simulink model "SIM_continuousFermenter"  (R2023b)
settings: Solver=VariableStepAuto  StartTime=0.0  StopTime=500  RelTol=1e-3
values from neighbouring files (symbols this model uses):
  Ts = 0.5    [NMPC_conFer.m]
libraries: sharedTrackingLibrary x1, mpclib x1, simulink x1, SignalEditorBlockLib x1
settings Model: Creator=akeebismail  LastModifiedBy=akeebismail

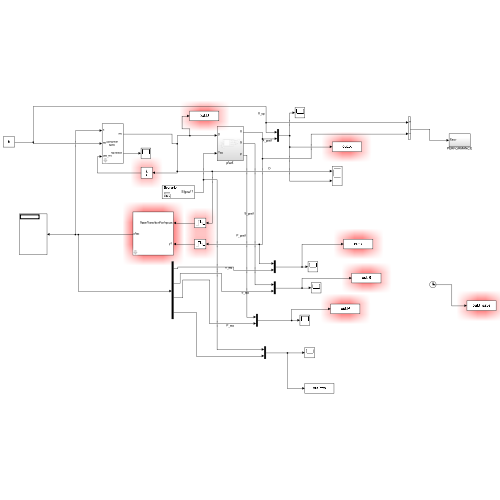
[thumbnail: Simulink's stored preview of the top-level diagram]
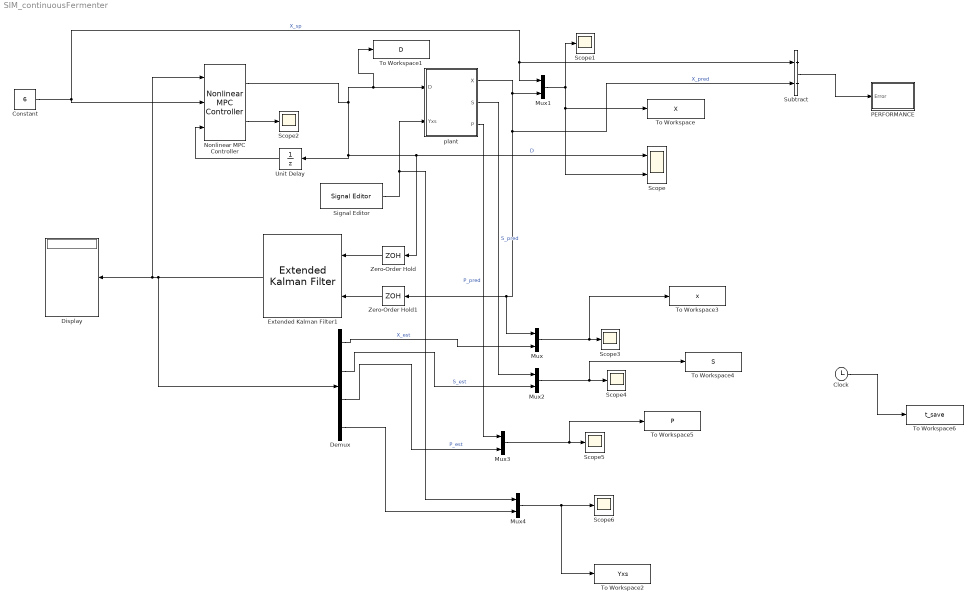
== system SIM_continuousFermenter ==
  Clock : Clock
  Constant : Constant  Value=6
  Demux : Demux
  Display : Display
  Extended Kalman Filter1 : sharedTrackingLibrary/Extended Kalman Filter  StateTransitionFcn=conFerStateFcnDT  HasStateTransitionJacobianFcn=off  HasAdditiveProcessNoise=Additive  ProcessNoise=[1e1;1e1;1e1;0.2]  HasTimeVaryingProcessNoise=off  HasStateTransitionFcnExtraArgument=1  InitialState=x0  InitialStateCovariance=[1;1;1;1]  MeasurementFcn1=conFerMeasFcn  HasMeasurementJacobianFcn1=off  HasMeasurementEnablePort1=off  HasAdditiveMeasurementNoise1=Additive  MeasurementNoise1=1e-3  HasTimeVaryingMeasurementNoise1=off  HasMeasurementFcnExtraArgument1=0  HasMeasurementWrapping1=off  MeasurementFcn2=myMeasurementFcn  HasMeasurementJacobianFcn2=off  HasMeasurementEnablePort2=off  HasAdditiveMeasurementNoise2=Additive  MeasurementNoise2=1  HasTimeVaryingMeasurementNoise2=off  HasMeasurementFcnExtraArgument2=0  HasMeasurementWrapping2=off  MeasurementFcn3=myMeasurementFcn  HasMeasurementJacobianFcn3=off  HasMeasurementEnablePort3=off  HasAdditiveMeasurementNoise3=Additive  MeasurementNoise3=1  HasTimeVaryingMeasurementNoise3=off  HasMeasurementFcnExtraArgument3=0  HasMeasurementWrapping3=off  MeasurementFcn4=myMeasurementFcn  HasMeasurementJacobianFcn4=off  HasMeasurementEnablePort4=off  HasAdditiveMeasurementNoise4=Additive  MeasurementNoise4=1  HasTimeVaryingMeasurementNoise4=off  HasMeasurementFcnExtraArgument4=0  HasMeasurementWrapping4=off  MeasurementFcn5=myMeasurementFcn  HasMeasurementJacobianFcn5=off  HasMeasurementEnablePort5=off  HasAdditiveMeasurementNoise5=Additive  MeasurementNoise5=1  HasTimeVaryingMeasurementNoise5=off  HasMeasurementFcnExtraArgument5=0  HasMeasurementWrapping5=off  EnableMultirate=off  StateTransitionFcnSampleTime=1  MeasurementFcn1SampleTime=1  MeasurementFcn2SampleTime=1  MeasurementFcn3SampleTime=1  MeasurementFcn4SampleTime=1  MeasurementFcn5SampleTime=1  UseCurrentEstimator=on  OutputStateCovariance=off  DataType=double  SampleTime=Ts  NumberOfMeasurements=1
  Mux{,1..4} (5 alike) : Mux  Inputs=2
  Nonlinear MPC Controller : mpclib/Nonlinear MPC Controller  nlmpcobj=nlobj  UseObjectTs=on  UseMEX=off  md_enabled=off  mvtarget_enabled=off  param_enabled=off  cost_enabled=off  mvseq_enabled=off  stateseq_enabled=off  ovseq_enabled=off  slack_enabled=off  status_enabled=on  ov_min=off  ov_max=off  mv_min=off  mv_max=off  mvrate_min=off  mvrate_max=off  state_min=off  state_max=off  ov_weight=off  mv_weight=off  mvrate_weight=off  ecr_weight=off  nlp_initialize=off
  PERFORMANCE : Subsystem
  Scope : Scope  NumInputPorts=2
  Scope{1..6} (6 alike) : Scope
  Signal Editor : SignalEditorBlockLib/Signal Editor  FileName=Yxs.mat  ActiveScenario=Scenario  ActiveSignal=Signal 1  IsBus=off  OutputBusObjectStr=Bus: BusObject  SampleTime=Ts  Interpolate=off  ZeroCross=off  OutputAfterFinalValue=Setting to zero  Unit=inherit  PreserveSignalName=on  ApplySigPropsToAllScenarios=on  ApplySigPropsToAllSignals=off
  Subtract : Sum  Inputs=+-
  To Workspace : ToWorkspace  VariableName=X  SaveFormat=Timeseries  SampleTime=Ts
  To Workspace1 : ToWorkspace  VariableName=D  SaveFormat=Timeseries  SampleTime=Ts
  To Workspace2 : ToWorkspace  VariableName=Yxs  SaveFormat=Timeseries  SampleTime=-1
  To Workspace3 : ToWorkspace  VariableName=x  SaveFormat=Timeseries  SampleTime=Ts
  To Workspace4 : ToWorkspace  VariableName=S  SaveFormat=Timeseries  SampleTime=Ts
  To Workspace5 : ToWorkspace  VariableName=P  SaveFormat=Timeseries  SampleTime=Ts
  To Workspace6 : ToWorkspace  VariableName=t_save  SaveFormat=Timeseries  SampleTime=Ts
  Unit Delay : UnitDelay  InitialCondition=0.202  SampleTime=Ts  HasFrameUpgradeWarning=on
  Zero-Order Hold : ZeroOrderHold  SampleTime=Ts
  Zero-Order Hold1 : ZeroOrderHold  SampleTime=Ts
  plant : Subsystem
  wires:
  Nonlinear MPC Controller/1 -> Zero-Order Hold/1, Scope/1, Unit Delay/1, To Workspace1/1, plant/1(D)  "D"
  Constant/1 -> Nonlinear MPC Controller/2, Subtract/1, Mux1/1  "X_sp"
  Nonlinear MPC Controller/2 -> Scope2/1
  plant/1(X) -> Subtract/2, Zero-Order Hold1/1, Mux/1, Mux1/2  "X_pred"
  Unit Delay/1 -> Nonlinear MPC Controller/3
  Mux1/1 -> Scope/2, To Workspace/1, Scope1/1
  Extended Kalman Filter1/1 -> Demux/1, Nonlinear MPC Controller/1, Display/1
  Zero-Order Hold/1 -> Extended Kalman Filter1/1
  Mux/1 -> To Workspace3/1, Scope3/1
  Demux/1 -> Mux/2  "X_est"
  Zero-Order Hold1/1 -> Extended Kalman Filter1/2
  Demux/3 -> Mux3/2  "P_est"
  Demux/2 -> Mux2/2  "S_est"
  plant/2(S) -> Mux2/1  "S_pred"
  plant/3(P) -> Mux3/1  "P_pred"
  Mux2/1 -> To Workspace4/1, Scope4/1
  Mux3/1 -> To Workspace5/1, Scope5/1
  Demux/4 -> Mux4/2
  Signal Editor/1 -> Mux4/1, plant/2(Yxs)
  Mux4/1 -> To Workspace2/1, Scope6/1
  Clock/1 -> To Workspace6/1
  Subtract/1 -> PERFORMANCE/1(Error)

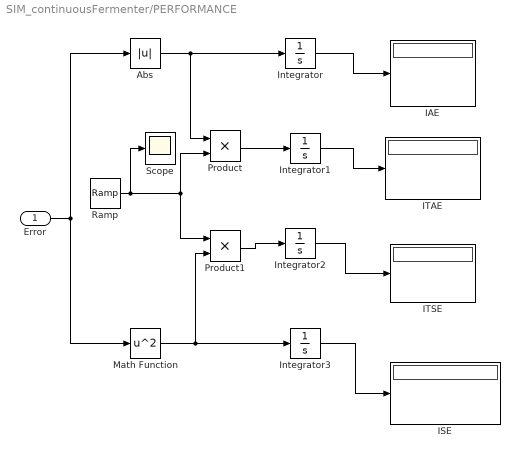
== system SIM_continuousFermenter/PERFORMANCE ==
  Error : Inport
  Abs : Abs  SaturateOnIntegerOverflow=off
  IAE : Display
  ISE : Display
  ITAE : Display
  ITSE : Display
  Integrator{,1..3} (4 alike) : Integrator
  Math Function : Math  Operator=square  SignedPower=on
  Product : Product  RndMeth=Zero
  Product1 : Product  RndMeth=Zero
  Ramp : simulink/Sources/Ramp  slope=1  start=0  InitialOutput=0
  Scope : Scope
  wires:
  Error/1 -> Math Function/1, Abs/1
  Abs/1 -> Integrator/1, Product/1
  Integrator/1 -> IAE/1
  Ramp/1 -> Product/2, Product1/1, Scope/1
  Math Function/1 -> Integrator3/1, Product1/2
  Product1/1 -> Integrator2/1
  Product/1 -> Integrator1/1
  Integrator3/1 -> ISE/1
  Integrator2/1 -> ITSE/1
  Integrator1/1 -> ITAE/1

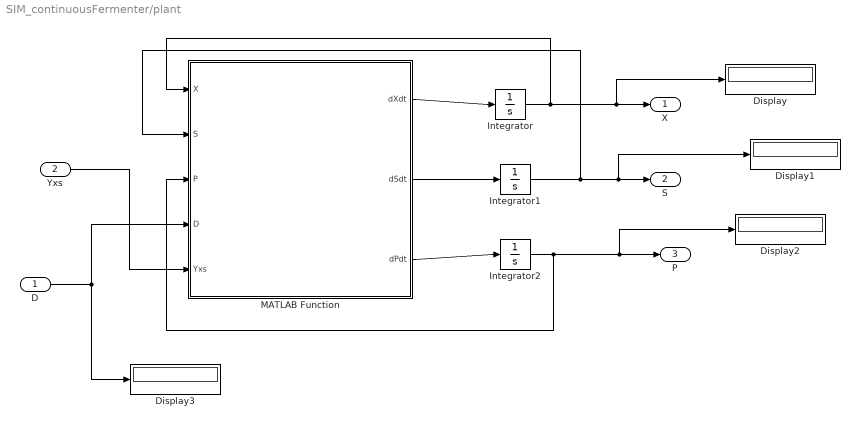
== system SIM_continuousFermenter/plant ==
  D : Inport
  Yxs : Inport  Port=2
  Display{,1..3} (4 alike) : Display
  Integrator : Integrator  InitialCondition=5
  Integrator1 : Integrator  InitialCondition=5
  Integrator2 : Integrator  InitialCondition=19.14
  MATLAB Function : MATLAB Function  TreatAsAtomicUnit=on
  X : Outport
  S : Outport  Port=2
  P : Outport  Port=3
  wires:
  MATLAB Function/1(dXdt) -> Integrator/1
  MATLAB Function/3(dPdt) -> Integrator2/1
  MATLAB Function/2(dSdt) -> Integrator1/1
  D/1 -> Display3/1, MATLAB Function/4(D)
  Integrator/1 -> Display/1, X/1, MATLAB Function/1(X)
  Integrator2/1 -> Display2/1, P/1, MATLAB Function/3(P)
  Integrator1/1 -> Display1/1, S/1, MATLAB Function/2(S)
  Yxs/1 -> MATLAB Function/5(Yxs)

== matlab function SIM_continuousFermenter/plant/MATLAB Function ==
  data: X input; dXdt output; S input; P input; D input; dSdt output; dPdt output; Yxs input
function [dXdt,dSdt,dPdt] = continuous_fermenter(X,S,P,D,Yxs)

values = {22,1.2,50,20,2.2,0.2,0.48};

[Ki,Km,Pm,Sf,alpha,beta,miu_m] = values{:};


miu = (miu_m * (1 - (P/Pm))) * S / (Km + S + (S^2 / Ki))  ;

dXdt = -D * X + miu * X     ;

dSdt = D * (Sf - S) - (1/Yxs) * miu * X   ;

dPdt = -D * P + (alpha * miu + beta) * X   ;

end
